simulink model "BLDC_EKF"  (R2024b)
settings: Solver=ode4  StartTime=0.0  StopTime=10.0  FixedStep=0.0001  RelTol=1e-3
values from neighbouring files (symbols this model uses):
  d = 0.35757    [DRBA_motor_EKF.m]    (also in DRBA_motor_PID_control.m; DRBA_motor_sysid.m = 0.1)
  dt = 0.005    [DRBA_motor_EKF.m]    (also in DRBA_motor_PID_control.m)
  f = 0.53378    [DRBA_motor_EKF.m]    (also in DRBA_motor_PID_control.m; DRBA_motor_sysid.m = 0.05)
  J = 0.05    [DRBA_motor_EKF.m]    (also in DRBA_motor_PID_control.m; DRBA_motor_sysid.m = 0.03)
  Kb = 20.91    [DRBA_motor_EKF.m]    (also in DRBA_motor_PID_control.m; DRBA_motor_sysid.m = 22)
  Kt = 0.7    [DRBA_motor_EKF.m]    (also in DRBA_motor_PID_control.m; DRBA_motor_sysid.m = 0.72)
  L = 0.00069    [DRBA_motor_EKF.m]    (also in DRBA_motor_PID_control.m; DRBA_motor_sysid.m = 0.00067)
  R = 0.0755    [DRBA_motor_EKF.m]    (also in DRBA_motor_PID_control.m; DRBA_motor_sysid.m = 0.0725)
settings Model: Creator=User  LastModifiedBy=User

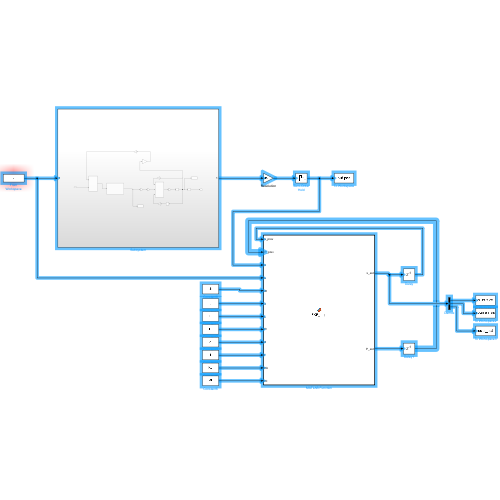
[thumbnail: Simulink's stored preview of the top-level diagram]
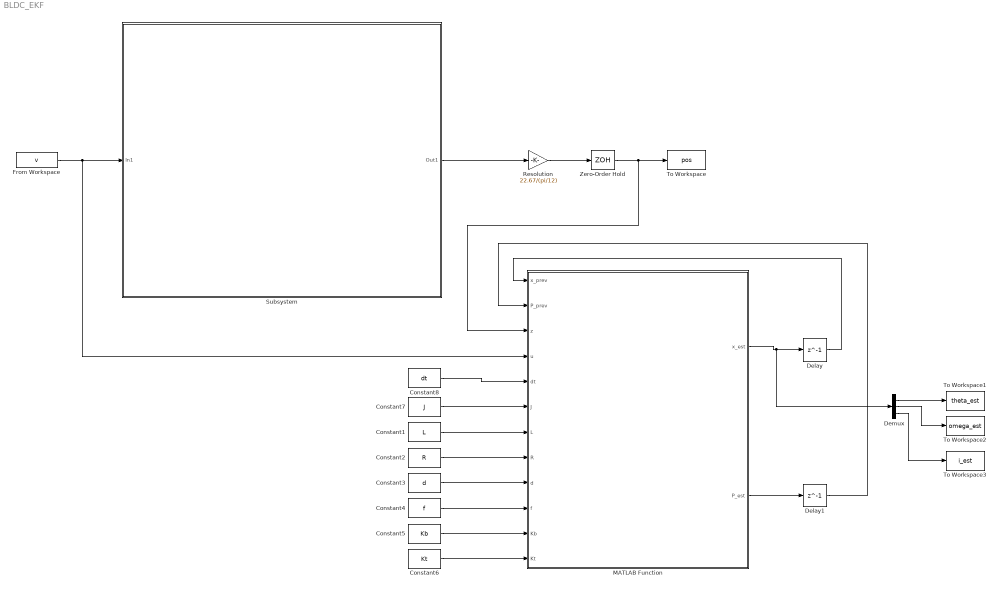
== system BLDC_EKF ==
  Constant1 : Constant  Value=L
  Constant2 : Constant  Value=R
  Constant3 : Constant  Value=d
  Constant4 : Constant  Value=f
  Constant5 : Constant  Value=Kb
  Constant6 : Constant  Value=Kt
  Constant7 : Constant  Value=J
  Constant8 : Constant  Value=dt
  Delay : Delay  DelayLength=1  InitialCondition=[0;0;0]
  Delay1 : Delay  DelayLength=1  InitialCondition=diag([0.01, 0.1, 1])
  Demux : Demux  Outputs=3
  From Workspace : FromWorkspace  VariableName=v
  MATLAB Function : MATLAB Function  TreatAsAtomicUnit=on  SystemSampleTime=0.005
  Resolution : Gain  Gain=22.67/(pi/12)  OutDataTypeStr=int32  RndMeth=Zero  SaturateOnIntegerOverflow=on
  Subsystem : Subsystem  SystemSampleTime=0.0001
  To Workspace : ToWorkspace  VariableName=pos  SampleTime=-1
  To Workspace1 : ToWorkspace  VariableName=theta_est  SampleTime=-1
      settings: Save2DSignal=2-D array (concatenate along first dimension)
  To Workspace2 : ToWorkspace  VariableName=omega_est  SampleTime=-1
      settings: Save2DSignal=2-D array (concatenate along first dimension)
  To Workspace3 : ToWorkspace  VariableName=i_est  SampleTime=-1
      settings: Save2DSignal=2-D array (concatenate along first dimension)
  Zero-Order Hold : ZeroOrderHold  SampleTime=0.005
  wires:
  Resolution/1 -> Zero-Order Hold/1
  From Workspace/1 -> MATLAB Function/4(u), Subsystem/1(In1)
  Subsystem/1(Out1) -> Resolution/1
  Zero-Order Hold/1 -> MATLAB Function/3(z), To Workspace/1
  Constant7/1 -> MATLAB Function/6(J)
  Constant1/1 -> MATLAB Function/7(L)
  Constant2/1 -> MATLAB Function/8(R)
  Constant3/1 -> MATLAB Function/9(d)
  Constant4/1 -> MATLAB Function/10(f)
  Constant5/1 -> MATLAB Function/11(Kb)
  Constant6/1 -> MATLAB Function/12(Kt)
  Constant8/1 -> MATLAB Function/5(dt)
  MATLAB Function/1(x_est) -> Demux/1, Delay/1
  Delay/1 -> MATLAB Function/1(x_prev)
  MATLAB Function/2(P_est) -> Delay1/1
  Delay1/1 -> MATLAB Function/2(P_prev)
  Demux/1 -> To Workspace1/1
  Demux/2 -> To Workspace2/1
  Demux/3 -> To Workspace3/1

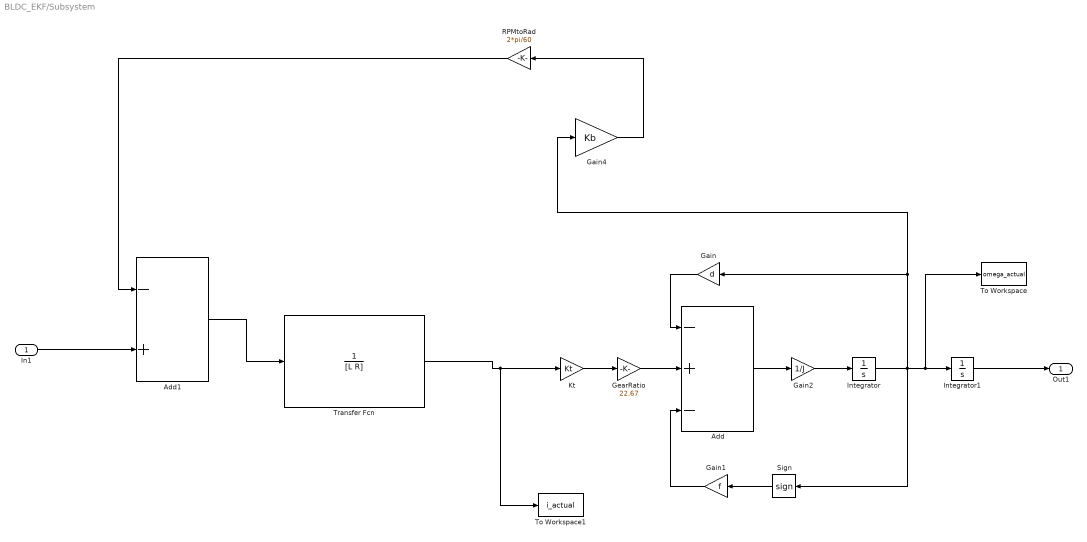
== system BLDC_EKF/Subsystem ==
  In1 : Inport
  Add : Sum  Inputs=-+-
  Add1 : Sum  Inputs=-+
  Gain : Gain  Gain=d
  Gain1 : Gain  Gain=f
  Gain2 : Gain  Gain=1/J
  Gain4 : Gain  Gain=Kb
  GearRatio : Gain  Gain=22.67
  Integrator : Integrator
  Integrator1 : Integrator
  Kt : Gain  Gain=Kt
  RPMtoRad : Gain  Gain=2*pi/60
  Sign : Signum  ZeroCross=off
  To Workspace : ToWorkspace  VariableName=omega_actual  SampleTime=-1
  To Workspace1 : ToWorkspace  VariableName=i_actual  SampleTime=-1
  Transfer Fcn : TransferFcn  Denominator=[L R]
  Out1 : Outport
  wires:
  Gain/1 -> Add/1
  Integrator1/1 -> Out1/1
  Kt/1 -> GearRatio/1
  GearRatio/1 -> Add/2
  RPMtoRad/1 -> Add1/1
  In1/1 -> Add1/2
  Gain2/1 -> Integrator/1
  Transfer Fcn/1 -> To Workspace1/1, Kt/1
  Integrator/1 -> To Workspace/1, Integrator1/1, Gain4/1, Gain/1, Sign/1
  Add/1 -> Gain2/1
  Add1/1 -> Transfer Fcn/1
  Gain1/1 -> Add/3
  Sign/1 -> Gain1/1
  Gain4/1 -> RPMtoRad/1

== matlab function BLDC_EKF/MATLAB Function ==
  data: x_prev input double size=[3 1]; P_prev input double size=[3 3]; z input; u input; x_est output double size=[3 1]; dt input; P_est output double size=[3 3]; J input; L input; R input; d input; f input; Kb input; Kt input
function [x_est, P_est] = EKF_step(x_prev,P_prev,z,u,dt,J,L,R,d,f,Kb,Kt)

x_est = zeros(3,1);
P_est = zeros(3,3);
z = double(z)*pi/12/22.67;

eps = 1/50;

% Previous state
theta = x_prev(1);
omega = x_prev(2);
i = x_prev(3);

% Nonlinear prediction
theta_pred = theta + omega*dt;
omega_pred = omega + 1/J*(Kt*22.67*i-d*omega-sign(omega)*f)*dt;
i_pred = i + 1/L*(u-R*i-Kb*omega*2*pi/60)*dt;

x_pred = [theta_pred;omega_pred;i_pred];

% Jacobian
d_friction_omega = f/eps*(1-tanh(omega/eps)^2);

F_k = [1, dt, 0;
       0, 1-dt/J*(d+d_friction_omega),dt/J*Kt*22.67;
       0, -dt/L*Kb*2*pi/60, 1-dt/L*R];

% Process noise
Q_n = diag([1e-5,1e-2,1e-1]);

P_pred = F_k*P_prev*F_k'+Q_n;

% Measurement
H_k = [1,0,0];
R_n = 0.001;

% Update
y = z - H_k*x_pred;
S = H_k*P_pred*H_k'+R_n;
K_k = P_pred*H_k'/S;

x_est = x_pred + K_k*y;
P_est = (eye(3)-K_k*H_k)*P_pred;
